simulink model "Simulink"  (R2021a)
settings: Solver=VariableStepAuto  StartTime=0.0  StopTime=50  RelTol=1e-3
libraries: commdigbbndam3 x2, commchan3 x1, commsink2 x1, phaseddetectlib x1, commrandsrc2 x1
settings Model: Creator=Mario  LastModifiedBy=Mario

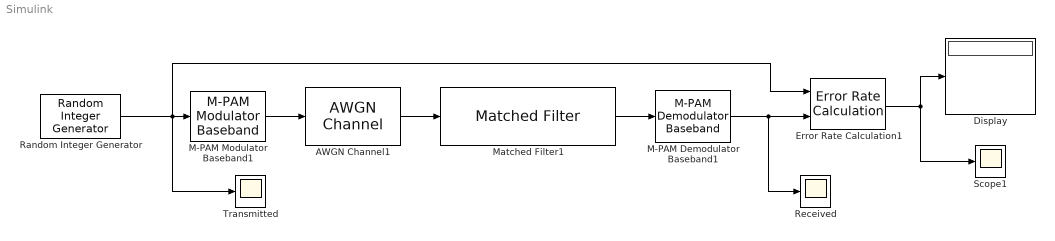
== system Simulink ==
  AWGN Channel1 : commchan3/AWGN Channel  InputProcessing=Columns as channels (frame based)  seed=67  noiseMode="Signal to noise ratio  (Eb/No)"  EbNodB=15  EsNodB=10  SNRdB=10  bitsPerSym=1  Ps=1  Tsym=1  variance=1
  Display : Display
  Error Rate Calculation1 : commsink2/Error Rate Calculation  N=0  st_delay=0  cp_mode=Entire frame  subframe=[]  PMode=Port  WsName=ErrorVec  RsMode2=off  stop=on  numErr=100  maxBits=1e6
  M-PAM Demodulator Baseband1 : commdigbbndam3/M-PAM Demodulator Baseband  M=8  OutType=Integer  Dec=Gray  PowType=Min. distance between symbols  MinDist=2  AvgPow=1  PeakPow=1  outDtype1=Inherit via internal rule  outDtype2=Inherit via internal rule  denormFactorWordLen=16  denormFactorDataTypeStr=Inherit: Same word length as input  denormFactorLastDataTypeStr=Inherit: Same word length as input  prodOutWordLen=16  prodOutRoundingMode=Floor  prodOutOverflowMode=Wrap  prodOutOvFlMode=off  prodOutOvFlModeLastStrValue=off  sumWordLen=16
      settings: SourceProductBaseCode=CM
  M-PAM Modulator Baseband1 : commdigbbndam3/M-PAM Modulator Baseband  M=8  InType=Integer  Enc=Gray  PowType=Min. distance between symbols  MinDist=2  AvgPow=1  PeakPow=1  outDtype=double  outWordLen=16  outUDDataType=sfix(16)  outFracLenMode=Best precision  outFracLen=15  outDataTypeStr=double  outLastDataTypeStr=double
      settings: SourceProductBaseCode=CM
  Matched Filter1 : phaseddetectlib/Matched Filter  CoefficientsSource=Property  Coefficients=[ 1; 1 ]  SpectrumWindow=None  CustomSpectrumWindow=@hamming  SpectrumRange=[ 0, 1e5 ]  SampleRateFromInputCheckbox=on  SampleRate=1e6  SidelobeAttenuation=30  Beta=0.5  Nbar=4  GainOutputPort=off  MaximumNumInputSamplesSource=Auto  MaximumNumInputSamples=100  SimulateUsing=Interpreted execution
      settings: SourceProductBaseCode=AR
  Random Integer Generator : commrandsrc2/Random Integer Generator  mul=8  seed=10  Ts=1  frameBased=off  sampPerFrame=1  orient=off  outDataType=double
      settings: SourceProductBaseCode=CM
  Received : Scope
  Scope1 : Scope
  Transmitted : Scope
  wires:
  M-PAM Modulator Baseband1/1 -> AWGN Channel1/1
  AWGN Channel1/1 -> Matched Filter1/1
  Matched Filter1/1 -> M-PAM Demodulator Baseband1/1
  Random Integer Generator/1 -> Error Rate Calculation1/1, M-PAM Modulator Baseband1/1, Transmitted/1
  M-PAM Demodulator Baseband1/1 -> Error Rate Calculation1/2, Received/1
  Error Rate Calculation1/1 -> Display/1, Scope1/1
